simulink model "ThreeTankOpen"  (R2024b)
settings: Solver=ode45  StartTime=0.0  StopTime=50  RelTol=1e-3  EnableMultiTasking=on
undefined symbols (not defined in the file): A, Atank, B, g, H, href, q11, q1ref, q21, q2ref, tUnit
settings Model: Creator=nmueller  LastModifiedBy=nachi
settings SolverCC: AlgebraicLoopSolver=TrustRegion
settings DataIOCC: LimitDataPoints=on  SaveFormat=Array  ReturnWorkspaceOutputs=off
settings OptimizationCC: LifeSpan=inf
settings DebuggingCC: SolverPrmCheckMsg=warning  UnconnectedInputMsg=warning  UnconnectedOutputMsg=warning  UnconnectedLineMsg=warning  SFUnexpectedBacktrackingDiag=warning  SFNoUnconditionalDefaultTransitionDiag=warning  SFExecutionAtInitializationDiag=none  ArithmeticOperatorsInVariantConditions=warning
settings HardwareCC: ProdBitPerPointer=32  ProdBitPerSizeT=32  ProdBitPerPtrDiffT=32  ProdLargestAtomicFloat=None  ProdIntDivRoundTo=Undefined  ProdEndianess=Unspecified  ProdWordSize=32  ProdHWDeviceType=32-bit Generic
settings ModelReferenceCC: PropagateSignalLabelsOutOfModel=off
settings SFSimCC: SimUseLocalCustomCode=off  CustomCodeUndefinedFunction=UseInterfaceOnly
settings RTWCC: RTWUseLocalCustomCode=off  GPUComputeCapability=3.5
settings CodeAppCC: StateflowObjectComments=on
settings GRTTargetCC: TargetLangStandard=C89/C90 (ANSI)
settings ConfigComp: CovMetricSettings=dw  CovSaveCumulativeToWorkspaceVar=on  CovSaveSingleToWorkspaceVar=on  CovExternalEMLEnable=off  CovSFcnEnable=off

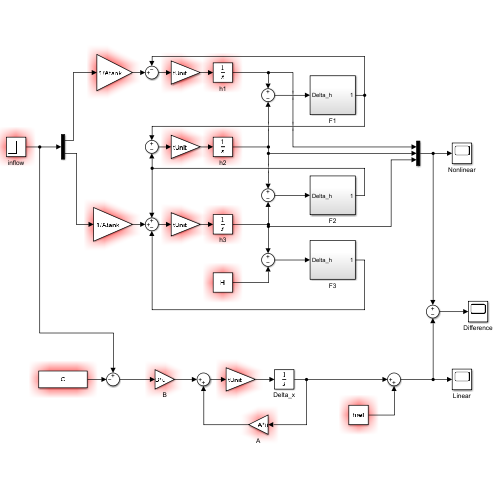
[thumbnail: Simulink's stored preview of the top-level diagram]
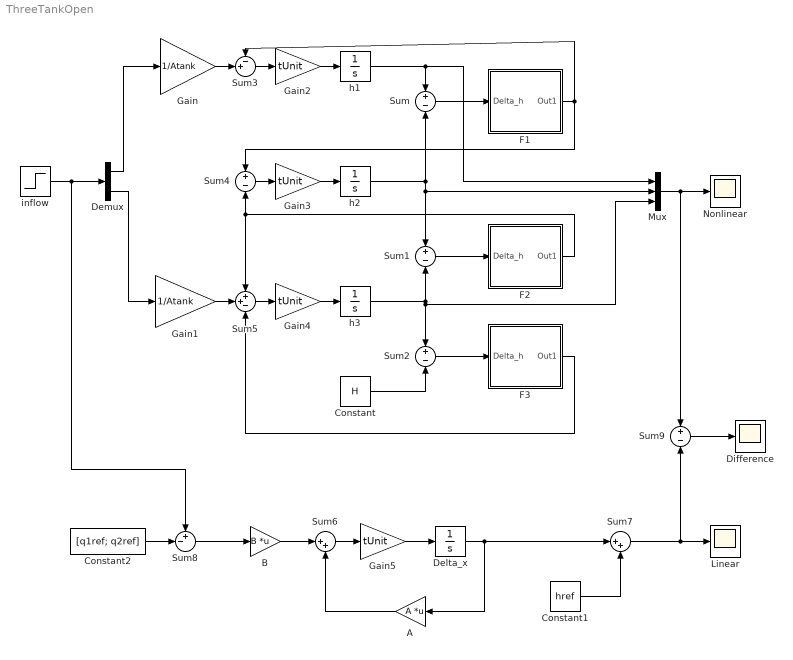
== system ThreeTankOpen ==
  A : Gain  Gain=A  Multiplication=Matrix(K*u)
  B : Gain  Gain=B  Multiplication=Matrix(K*u)
  Constant : Constant  Value=H
  Constant1 : Constant  Value=href
  Constant2 : Constant  Value=[q1ref; q2ref]
  Delta_x : Integrator  InitialCondition=[ 0; 0; 0 ]
  Demux : Demux  Outputs=2
  Difference : Scope
  F1 : Subsystem
  F2 : Subsystem
  F3 : Subsystem
  Gain : Gain  Gain=1/Atank
  Gain1 : Gain  Gain=1/Atank
  Gain{2..5} (4 alike) : Gain  Gain=tUnit
  Linear : Scope
  Mux : Mux  Inputs=3
  Nonlinear : Scope
  Sum{,1..2,4,9} (5 alike) : Sum  Inputs=+-
  Sum3 : Sum  Inputs=-+|
  Sum5 : Sum  Inputs=++-
  Sum6 : Sum  Inputs=|++
  Sum7 : Sum  Inputs=|++
  Sum8 : Sum  Inputs=+-|
  h1 : Integrator  InitialCondition=href(1)
  h2 : Integrator  InitialCondition=href(2)
  h3 : Integrator  InitialCondition=href(3)
  inflow : Step  Before=[q1ref;q2ref]  After=[q11;q21]  SampleTime=0
  wires:
  h1/1 -> Mux/1, Sum/1
  h2/1 -> Sum/2, Mux/2, Sum1/1
  Sum/1 -> F1/1(Delta_h)
  h3/1 -> Sum1/2, Mux/3, Sum2/1
  Sum1/1 -> F2/1(Delta_h)
  Constant/1 -> Sum2/2
  Sum2/1 -> F3/1(Delta_h)
  Demux/1 -> Gain/1
  Demux/2 -> Gain1/1
  F1/1(Out1) -> Sum4/1, Sum3/1
  Gain/1 -> Sum3/2
  Sum3/1 -> Gain2/1
  Sum4/1 -> Gain3/1
  F2/1(Out1) -> Sum4/2, Sum5/1
  Gain1/1 -> Sum5/2
  F3/1(Out1) -> Sum5/3
  Sum5/1 -> Gain4/1
  Mux/1 -> Sum9/1, Nonlinear/1
  Sum6/1 -> Gain5/1
  Delta_x/1 -> Sum7/1, A/1
  A/1 -> Sum6/2
  B/1 -> Sum6/1
  Constant1/1 -> Sum7/2
  Sum7/1 -> Sum9/2, Linear/1
  Constant2/1 -> Sum8/2
  inflow/1 -> Sum8/1, Demux/1
  Sum8/1 -> B/1
  Gain2/1 -> h1/1
  Gain3/1 -> h2/1
  Gain4/1 -> h3/1
  Gain5/1 -> Delta_x/1
  Sum9/1 -> Difference/1

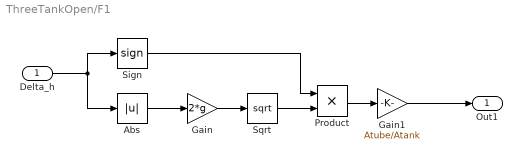
== system ThreeTankOpen/F1 ==
  Delta_h : Inport
  Abs : Abs  SaturateOnIntegerOverflow=off
  Gain : Gain  Gain=2*g
  Gain1 : Gain  Gain=Atube/Atank
  Product : Product
  Sign : Signum
  Sqrt : Sqrt
  Out1 : Outport
  wires:
  Product/1 -> Gain1/1
  Gain1/1 -> Out1/1
  Sign/1 -> Product/1
  Sqrt/1 -> Product/2
  Delta_h/1 -> Abs/1, Sign/1
  Abs/1 -> Gain/1
  Gain/1 -> Sqrt/1

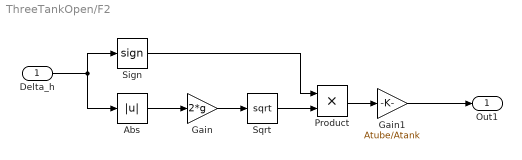
== system ThreeTankOpen/F2 ==
  Delta_h : Inport
  Abs : Abs  SaturateOnIntegerOverflow=off
  Gain : Gain  Gain=2*g
  Gain1 : Gain  Gain=Atube/Atank
  Product : Product
  Sign : Signum
  Sqrt : Sqrt
  Out1 : Outport
  wires:
  Gain/1 -> Sqrt/1
  Abs/1 -> Gain/1
  Delta_h/1 -> Sign/1, Abs/1
  Sqrt/1 -> Product/2
  Sign/1 -> Product/1
  Gain1/1 -> Out1/1
  Product/1 -> Gain1/1

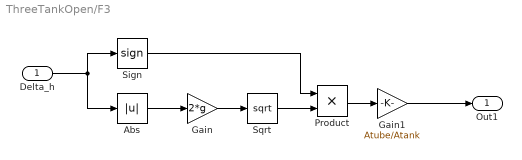
== system ThreeTankOpen/F3 ==
  Delta_h : Inport
  Abs : Abs  SaturateOnIntegerOverflow=off
  Gain : Gain  Gain=2*g
  Gain1 : Gain  Gain=Atube/Atank
  Product : Product
  Sign : Signum
  Sqrt : Sqrt
  Out1 : Outport
  wires:
  Product/1 -> Gain1/1
  Gain1/1 -> Out1/1
  Sign/1 -> Product/1
  Sqrt/1 -> Product/2
  Delta_h/1 -> Abs/1, Sign/1
  Abs/1 -> Gain/1
  Gain/1 -> Sqrt/1
